simulink model "Controlo_Atitude"  (R2020a)
settings: Solver=VariableStepAuto  StartTime=0.0  StopTime=60  RelTol=1e-3
values from neighbouring files (symbols this model uses):
  A = [Ybb  Yp+W0/U0      Yr-1  (g*cos(tt0))/U0 ... (first row only)    [Aterragem_sematuadores.m]    (also in EKC39.m)
  B = [YdA      YdR ... (first row only)    [Aterragem_sematuadores.m]    (also in EKC39.m)
  C = eye(4)    [Aterragem_sematuadores.m]    (also in EKC39.m)
  D = zeros(4,2)    [Aterragem_sematuadores.m]    (also in EKC39.m)
  k_integrativo2 = k_lqr(:,5:6)    [EKC39.m]
  k_interior2 = k_lqr(:,2:3)    [EKC39.m]
  k_proporcional2 = [k_lqr(:,1) k_lqr(:,4)]    [EKC39.m]
settings Model: Creator=vicen  LastModifiedBy=vicen

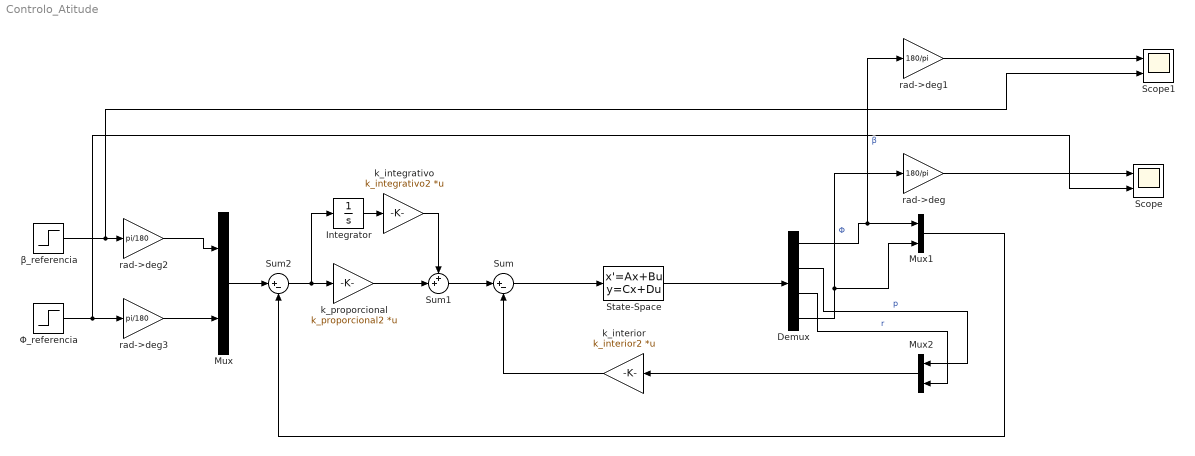
== system Controlo_Atitude ==
  Demux : Demux
  Integrator : Integrator
  Mux : Mux  Inputs=2
  Mux1 : Mux  Inputs=2
  Mux2 : Mux  Inputs=2
  Scope : Scope  NumInputPorts=2
  Scope1 : Scope  NumInputPorts=2
  State-Space : StateSpace  A=A  B=B  C=C  D=D  InitialCondition=0
  Sum : Sum  Inputs=|+-
  Sum1 : Sum  Inputs=++|
  Sum2 : Sum  Inputs=|+-
  k_integrativo : Gain  Gain=k_integrativo2  Multiplication=Matrix(K*u)
  k_interior : Gain  Gain=k_interior2  Multiplication=Matrix(K*u)
  k_proporcional : Gain  Gain=k_proporcional2  Multiplication=Matrix(K*u)
  rad->deg : Gain  Gain=180/pi
  rad->deg1 : Gain  Gain=180/pi
  rad->deg2 : Gain  Gain=pi/180
  rad->deg3 : Gain  Gain=pi/180
  Φ_referencia : Step  Time=20  After=10  SampleTime=0
  β_referencia : Step  Time=5  After=5  SampleTime=0
  wires:
  Sum/1 -> State-Space/1
  k_interior/1 -> Sum/2
  State-Space/1 -> Demux/1
  β_referencia/1 -> Scope1/2, rad->deg2/1
  k_integrativo/1 -> Sum1/1
  Integrator/1 -> k_integrativo/1
  k_proporcional/1 -> Sum1/2
  Sum2/1 -> Integrator/1, k_proporcional/1
  Mux/1 -> Sum2/1
  Φ_referencia/1 -> rad->deg3/1, Scope/2
  Demux/1 -> rad->deg1/1, Mux1/1  "β"
  Demux/2 -> Mux2/1  "p"
  Demux/3 -> Mux2/2  "r"
  Mux2/1 -> k_interior/1
  Demux/4 -> rad->deg/1, Mux1/2  "Φ"
  Mux1/1 -> Sum2/2
  Sum1/1 -> Sum/1
  rad->deg/1 -> Scope/1
  rad->deg1/1 -> Scope1/1
  rad->deg3/1 -> Mux/2
  rad->deg2/1 -> Mux/1
